simulink model "test"  (Simulink 8.0)
settings: Solver=FixedStepDiscrete  StartTime=0.0  StopTime=Inf  FixedStep=.001  RelTol=1e-3
CloseFcn:
  | rtwprivate ssgencode ModelCloseRequest rwalk_multi_local_v1
settings Model: Creator=limblab  LastModifiedBy=system administrator  ParamWorkspaceSource=ReferencedWorkspace  ExtModeArmWhenConnect=off  BufferReuse=off
settings DataIOCC: LimitDataPoints=off  SaveFormat=StructureWithTime  SignalLoggingSaveFormat=ModelDataLogs  SaveState=on  SignalLoggingName=sigsOut
settings OptimizationCC: BlockReduction=off  BooleanDataType=off  OptimizeBlockIOStorage=off  BufferReuse=off  ExpressionFolding=off  FoldNonRolledExpr=off  LocalBlockOutputs=off  InitFltsAndDblsToZero=on
settings DebuggingCC: SaveWithParameterizedLinksMsg=none  SignalResolutionControl=TryResolveAllWithWarning  SolverPrmCheckMsg=none  MultiTaskDSMMsg=warning  MultiTaskCondExecSysMsg=none  FcnCallInpInsideContextMsg=UseLocalSettings  StrictBusMsg=None
settings HardwareCC: ProdIntDivRoundTo=Zero  ProdEndianess=LittleEndian  ProdHWDeviceType=Generic->32-bit x86 compatible  TargetIntDivRoundTo=Floor  TargetEndianess=LittleEndian  TargetHWDeviceType=32-bit xPC Target (Intel Pentium)
settings SFSimCC: SimParseCustomCode=off
settings RTWCC: SystemTargetFile=xpctarget.tlc  TemplateMakefile=xpc_default_tmf  Description=xPC Target  GenerateReport=on  ProcessScript=xpctarget_make_rtw_hook  IncludeERTFirstTime=on  RTWCompilerOptimization=On
settings xpcTargetCC: TargetFcnLib=ansi_tfl_tmw.mat  CodeReplacementLibrary=XPC_BLAS  ParMdlRefBuildCompliant=on  ConcurrentExecutionCompliant=on  CombineSignalStateStructs=off  GRTInterface=on  xPCTaskExecutionProfile=off  xPCRL32EventNumber=5000  xPCisDownloadable=off  xPCLoadParamSetFile=off  xPCConcurrentTasks=off  xPCEnableSFAnimation=off

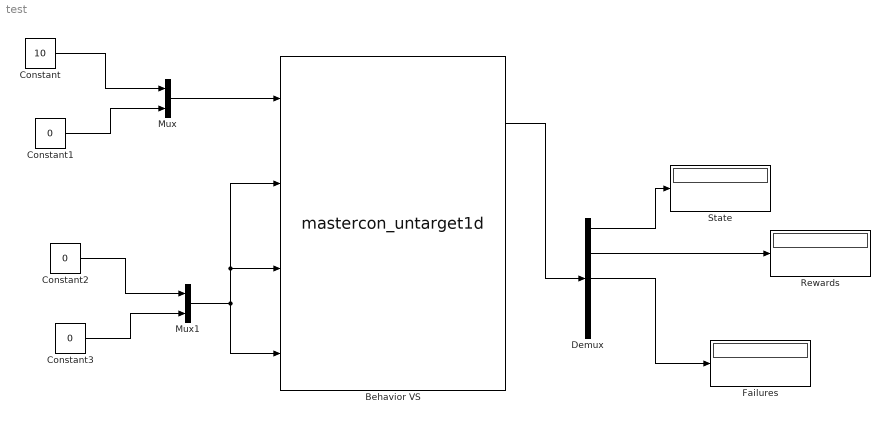
== system test ==
  Behavior VS : S-Function  FunctionName=mastercon_untarget1d  Parameters=1 0.5 1 0.5 1 0.5 1 1 3 1 90 10 2 3 3 2 1 5 8 1 2 3 4 0.25 0.25 0.25 0.25 0 0.2 7 3 5 0.2 0 1 5  EnableBusSupport=off
      mask Display:
      | disp('Master Control')
      | port_label('input',1,'pos')
      | port_label('input',2,'offsets')
      | port_label('input',3,'force')
      | port_label('input',4,'catch force')
      | port_label('output',1,'force')
      | port_label('output',2,'status')
      | port_label('output',3,'word')
      | port_label('output',4,'targets')
      | port_label('output',5,'reward')
      | port_label('output',6,'tone')
      | port_label('output',7,'version')
      | port_label('output',8,'pos')
  Constant : Constant  Value=10
  Constant1 : Constant  Value=0
  Constant2 : Constant  Value=0
  Constant3 : Constant  Value=0
  Demux : Demux  Outputs=5
  Failures : Display
  Mux : Mux  Inputs=2
  Mux1 : Mux  Inputs=2
  Rewards : Display
  State : Display
  wires:
  Constant/1 -> Mux/1
  Constant1/1 -> Mux/2
  Mux/1 -> Behavior VS/1
  Behavior VS/2 -> Demux/1
  Demux/1 -> State/1
  Constant2/1 -> Mux1/1
  Constant3/1 -> Mux1/2
  Mux1/1 -> Behavior VS/2, Behavior VS/3, Behavior VS/4
  Demux/2 -> Rewards/1
  Demux/3 -> Failures/1
